simulink model "rl_top_9bus"  (Simulink 10.3)
settings: Solver=ode113  StartTime=0.0  StopTime=2  RelTol=1e-3
libraries: simulink x9, rllib x1
settings Model: Creator=z0034ktr  LastModifiedBy=User  MultithreadedSim=on
settings DataIOCC: SignalLoggingSaveFormat=Dataset
settings OptimizationCC: ExpressionDepthLimit=128  LifeSpan=auto
settings DebuggingCC: UnderspecifiedInitializationDetection=Simplified  MergeDetectMultiDrivingBlocksExec=error  FcnCallInpInsideContextMsg=error  StateNameClashWarn=none  SFUnexpectedBacktrackingDiag=error  SFNoUnconditionalDefaultTransitionDiag=error  SFExecutionAtInitializationDiag=warning  ArithmeticOperatorsInVariantConditions=error
settings HardwareCC: ProdBitPerPointer=64  ProdBitPerSizeT=64  ProdBitPerPtrDiffT=64  ProdLargestAtomicFloat=Float  ProdIntDivRoundTo=Zero  ProdEndianess=LittleEndian  ProdWordSize=64  ProdHWDeviceType=Intel->x86-64 (Windows64)
settings ModelReferenceCC: PropagateSignalLabelsOutOfModel=on
settings SFSimCC: SimUseLocalCustomCode=on  CustomCodeUndefinedFunction=FilterOut
settings RTWCC: RTWUseLocalCustomCode=on
settings CodeAppCC: StateflowObjectComments=off
settings GRTTargetCC: TargetLangStandard=C99 (ISO)  CombineOutputUpdateFcns=on  GRTInterface=off
settings ConfigComp: CovMetricSettings=dwe  CovSaveCumulativeToWorkspaceVar=off  CovSaveSingleToWorkspaceVar=off  CovExternalEMLEnable=on

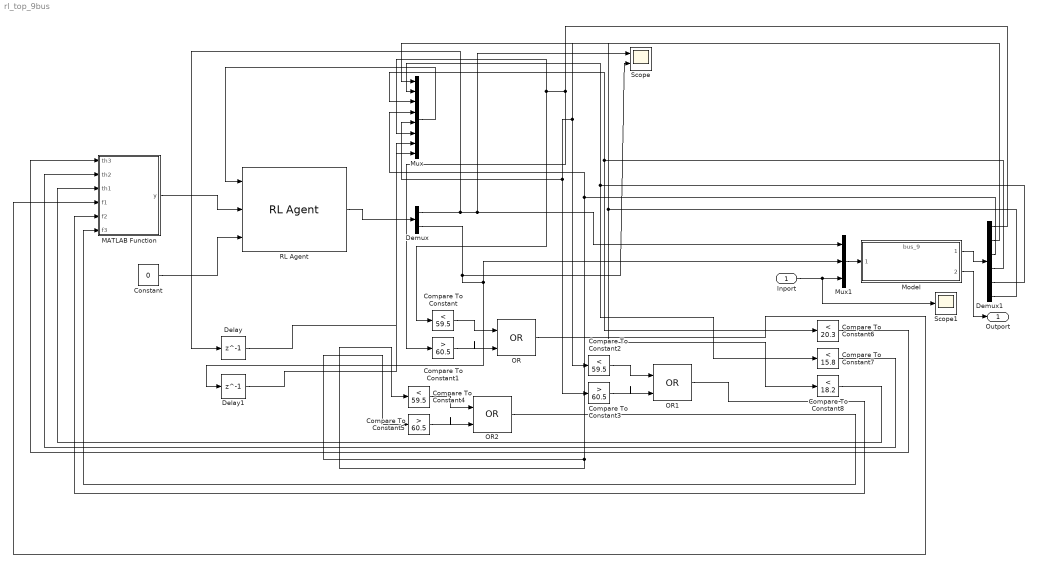
== system rl_top_9bus ==
  Inport : Inport
  Compare To Constant : simulink/Logic and Bit Operations/Compare To Constant  relop=<  const=59.5  OutDataTypeStr=boolean
  Compare To Constant1 : simulink/Logic and Bit Operations/Compare To Constant  relop=>  const=60.5  OutDataTypeStr=boolean
  Compare To Constant2 : simulink/Logic and Bit Operations/Compare To Constant  relop=<  const=59.5  OutDataTypeStr=boolean
  Compare To Constant3 : simulink/Logic and Bit Operations/Compare To Constant  relop=>  const=60.5  OutDataTypeStr=boolean
  Compare To Constant4 : simulink/Logic and Bit Operations/Compare To Constant  relop=<  const=59.5  OutDataTypeStr=boolean
  Compare To Constant5 : simulink/Logic and Bit Operations/Compare To Constant  relop=>  const=60.5  OutDataTypeStr=boolean
  Compare To Constant6 : simulink/Logic and Bit Operations/Compare To Constant  relop=<  const=20.3  OutDataTypeStr=boolean
  Compare To Constant7 : simulink/Logic and Bit Operations/Compare To Constant  relop=<  const=15.8  OutDataTypeStr=boolean
  Compare To Constant8 : simulink/Logic and Bit Operations/Compare To Constant  relop=<  const=18.2  OutDataTypeStr=boolean
  Constant : Constant  Value=0
  Delay : Delay  DelayLength=1
  Delay1 : Delay  DelayLength=1
  Demux : Demux  Outputs=2
  Demux1 : Demux  Outputs=6
  MATLAB Function : MATLAB Function  TreatAsAtomicUnit=on
  Model : ModelReference  ModelNameDialog=bus_9.mdl  SimulationMode=Normal  ModelReferenceVersion=1.16
  Mux : Mux  Inputs=8
  Mux1 : Mux  Inputs=3
  OR : Logic  Operator=OR  IconShape=distinctive  AllPortsSameDT=off  OutDataTypeStr=boolean
  OR1 : Logic  Operator=OR  IconShape=distinctive  AllPortsSameDT=off  OutDataTypeStr=boolean
  OR2 : Logic  Operator=OR  IconShape=distinctive  AllPortsSameDT=off  OutDataTypeStr=boolean
  RL Agent : rllib/RL Agent  Agent=agent9busnew2  ExternalActionAsInput=off  ProvideCumRwd=off  TreatAsDirectFeedthrough=on
  Scope : Scope  NumInputPorts=2
  Scope1 : Scope
  Outport : Outport
  wires:
  RL Agent/1 -> Demux/1
  Demux/1 -> Delay/1, Mux1/1, Scope/1
  Demux/2 -> Scope/2, Mux1/2, Delay1/1
  Mux/1 -> RL Agent/1
  Demux1/6 -> Compare To Constant8/1, Mux/1
  Demux1/5 -> Compare To Constant7/1, Mux/2
  Demux1/4 -> Compare To Constant6/1, Mux/3
  Demux1/1 -> Compare To Constant1/1, Compare To Constant/1, Mux/6
  Constant/1 -> RL Agent/3
  Compare To Constant/1 -> OR/1
  Compare To Constant1/1 -> OR/2
  Compare To Constant3/1 -> OR1/2
  Demux1/2 -> Compare To Constant3/1, Mux/5, Compare To Constant2/1
  Compare To Constant2/1 -> OR1/1
  Compare To Constant5/1 -> OR2/2
  Demux1/3 -> Mux/4, Compare To Constant5/1, Compare To Constant4/1
  Compare To Constant4/1 -> OR2/1
  Compare To Constant6/1 -> MATLAB Function/1(th3)
  Compare To Constant7/1 -> MATLAB Function/2(th2)
  Compare To Constant8/1 -> MATLAB Function/3(th1)
  OR/1 -> MATLAB Function/4(f1)
  OR1/1 -> MATLAB Function/5(f2)
  OR2/1 -> MATLAB Function/6(f3)
  Delay/1 -> Mux/7
  Delay1/1 -> Mux/8
  MATLAB Function/1(y) -> RL Agent/2
  Inport/1 -> Scope1/1, Mux1/3
  Mux1/1 -> Model/1
  Model/1 -> Demux1/1
  Model/2 -> Outport/1

== matlab function MATLAB Function ==
  data: th3 input double; th2 input double; th1 input double; f1 input double; f2 input double; y output double; f3 input double
function y = fcn(th3, th2, th1, f1, f2, f3)
w1=7;
w2=5;
w3=3;
rwd= (w1*(f1*th1)+w2*(f2*th2)+w3*(f3*th3));
y = rwd;
